simulink model "Add"  (R2015a)
settings: Solver=FixedStepDiscrete  SolverMode=SingleTasking  StartTime=0.0  StopTime=10.0  RelTol=1e-3
settings Model: CovMetricSettings=dwe  CovHtmlReporting=off  covSaveCumulativeToWorkspaceVar=off  CovSaveSingleToWorkspaceVar=off  CovExternalEMLEnable=on  Creator=hbourbou  LastModifiedBy=hbourbou
settings DataIOCC: LimitDataPoints=off  SaveFormat=Dataset
settings DebuggingCC: SFUnexpectedBacktrackingDiag=error  SFNoUnconditionalDefaultTransitionDiag=error
settings HardwareCC: ProdBitPerPointer=64  ProdLargestAtomicFloat=Float  ProdIntDivRoundTo=Zero  ProdEndianess=LittleEndian  ProdHWDeviceType=Specified
settings ModelReferenceCC: PropagateSignalLabelsOutOfModel=on
settings GRTTargetCC: TargetLangStandard=C99 (ISO)  GeneratePreprocessorConditionals=Use local settings

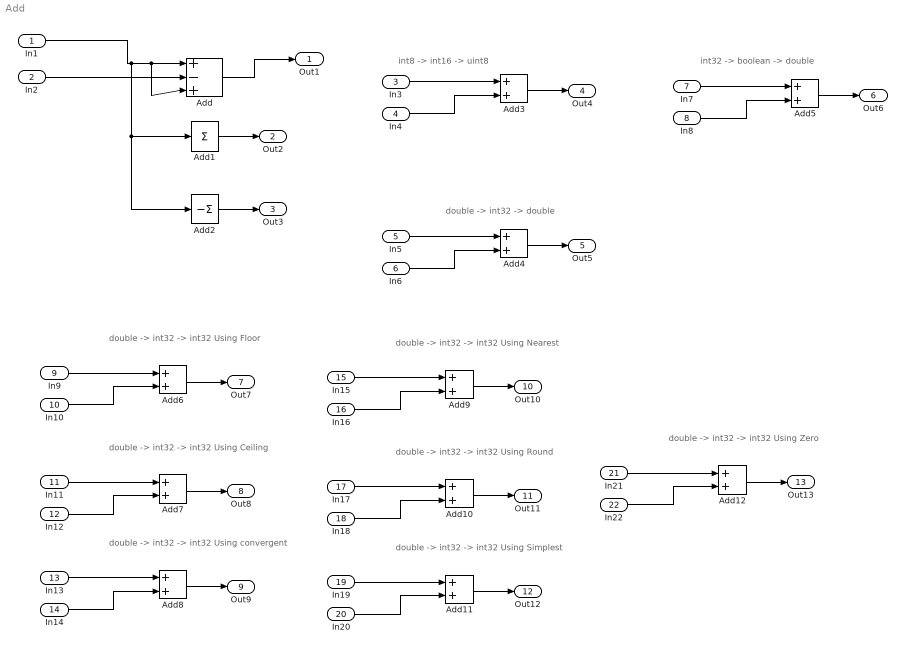
== system Add ==
  note: int8 -> int16 -> uint8
  note: int32 -> boolean -> double
  note: double -> int32 -> double
  note: double -> int32 -> int32 Using Floor
  note: double -> int32 -> int32 Using Ceiling
  note: double -> int32 -> int32 Using convergent
  note: double -> int32 -> int32 Using Round
  note: double -> int32 -> int32 Using Simplest
  note: double -> int32 -> int32 Using Nearest
  note: double -> int32 -> int32 Using Zero
  In1 : Inport  PortDimensions=3
  In2 : Inport  Port=2  PortDimensions=1
  In3 : Inport  Port=3  OutDataTypeStr=int8
  In4 : Inport  Port=4  OutDataTypeStr=int16
  In5 : Inport  Port=5  OutDataTypeStr=double
  In6 : Inport  Port=6  OutDataTypeStr=int32
  In7 : Inport  Port=7  OutDataTypeStr=int32
  In8 : Inport  Port=8  OutDataTypeStr=boolean
  In9 : Inport  Port=9  OutDataTypeStr=double
  In10 : Inport  Port=10  OutDataTypeStr=int32
  In11 : Inport  Port=11  OutDataTypeStr=double
  In12 : Inport  Port=12  OutDataTypeStr=int32
  In13 : Inport  Port=13  OutDataTypeStr=double
  In14 : Inport  Port=14  OutDataTypeStr=int32
  In15 : Inport  Port=15  OutDataTypeStr=double
  In16 : Inport  Port=16  OutDataTypeStr=int32
  In17 : Inport  Port=17  OutDataTypeStr=double
  In18 : Inport  Port=18  OutDataTypeStr=int32
  In19 : Inport  Port=19  OutDataTypeStr=double
  In20 : Inport  Port=20  OutDataTypeStr=int32
  In21 : Inport  Port=21  OutDataTypeStr=double
  In22 : Inport  Port=22  OutDataTypeStr=int32
  Add : Sum  Inputs=+|-|+
  Add1 : Sum  Inputs=+
  Add10 : Sum  AccumDataTypeStr=int32  OutDataTypeStr=int32  RndMeth=Round
  Add11 : Sum  AccumDataTypeStr=int32  OutDataTypeStr=int32  RndMeth=Simplest
  Add12 : Sum  AccumDataTypeStr=int32  OutDataTypeStr=int32  RndMeth=Zero
  Add2 : Sum  Inputs=-
  Add3 : Sum  AccumDataTypeStr=uint8  OutDataTypeStr=uint8
  Add4 : Sum  AccumDataTypeStr=double  OutDataTypeStr=double
  Add5 : Sum  AccumDataTypeStr=double  OutDataTypeStr=double
  Add6 : Sum  AccumDataTypeStr=int32  OutDataTypeStr=int32
  Add7 : Sum  AccumDataTypeStr=int32  OutDataTypeStr=int32  RndMeth=Ceiling
  Add8 : Sum  AccumDataTypeStr=int32  OutDataTypeStr=int32  RndMeth=Convergent
  Add9 : Sum  AccumDataTypeStr=int32  OutDataTypeStr=int32  RndMeth=Nearest
  Out1 : Outport
  Out2 : Outport  Port=2
  Out3 : Outport  Port=3
  Out4 : Outport  Port=4  OutDataTypeStr=uint8
  Out5 : Outport  Port=5
  Out6 : Outport  Port=6
  Out7 : Outport  Port=7
  Out8 : Outport  Port=8
  Out9 : Outport  Port=9
  Out10 : Outport  Port=10
  Out11 : Outport  Port=11
  Out12 : Outport  Port=12
  Out13 : Outport  Port=13
  wires:
  In2/1 -> Add/2
  Add/1 -> Out1/1
  Add1/1 -> Out2/1
  In1/1 -> Add2/1, Add1/1, Add/3, Add/1
  Add2/1 -> Out3/1
  Add3/1 -> Out4/1
  In3/1 -> Add3/1
  In4/1 -> Add3/2
  Add4/1 -> Out5/1
  In6/1 -> Add4/2
  In5/1 -> Add4/1
  Add5/1 -> Out6/1
  In8/1 -> Add5/2
  In7/1 -> Add5/1
  In10/1 -> Add6/2
  Add6/1 -> Out7/1
  In9/1 -> Add6/1
  In11/1 -> Add7/1
  Add7/1 -> Out8/1
  In12/1 -> Add7/2
  In13/1 -> Add8/1
  Add8/1 -> Out9/1
  In14/1 -> Add8/2
  Add11/1 -> Out12/1
  In18/1 -> Add10/2
  Add10/1 -> Out11/1
  In20/1 -> Add11/2
  In19/1 -> Add11/1
  In17/1 -> Add10/1
  In15/1 -> Add9/1
  Add9/1 -> Out10/1
  In16/1 -> Add9/2
  In22/1 -> Add12/2
  In21/1 -> Add12/1
  Add12/1 -> Out13/1
